simulink model "FSK_SIM"  (R2024a)
settings: Solver=VariableStepAuto  StartTime=0.0  StopTime=10.0  RelTol=1e-3
settings Model: Creator=adity  LastModifiedBy=adity

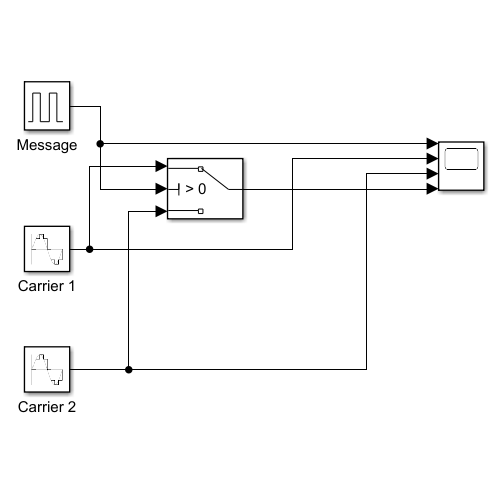
[thumbnail: Simulink's stored preview of the top-level diagram]
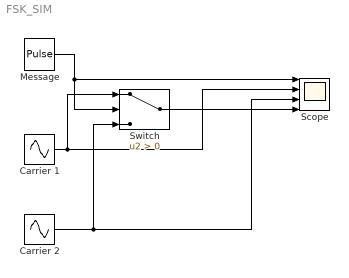
== system FSK_SIM ==
  Carrier 1 : Sin  Frequency=2*pi*50  SampleTime=1/1000000  VectorParams1D=off
  Carrier 2 : Sin  Frequency=2*pi*10  SampleTime=1/1000000  VectorParams1D=off
  Message : DiscretePulseGenerator  PulseType=Time based  Period=0.5  PulseWidth=50
  Scope : Scope  NumInputPorts=4
  Switch : Switch  Criteria=u2 > Threshold  SaturateOnIntegerOverflow=off  InputSameDT=off
  wires:
  Message/1 -> Switch/2, Scope/1
  Carrier 1/1 -> Switch/1, Scope/2
  Carrier 2/1 -> Scope/3, Switch/3
  Switch/1 -> Scope/4
